simulink model "fig10_70"  (Simulink 7.0)
settings: Solver=ode23s  SolverMode=SingleTasking  StartTime=0.0  StopTime=100.0  RelTol=1e-3  AbsTol=1e-6
values from neighbouring files (symbols this model uses):
  a = [f, 0*f ... (first row only)    [fig10_18.m]    (also in fig10_19.m; fig10_20.m; fig10_21.m; fig10_22.m)
  b = [g;0*g]    [fig10_18.m]    (also in fig10_19.m; fig10_20.m; fig10_21.m; fig10_22.m)
  c = [0*h, g']    [fig10_18.m]    (also in fig10_19.m; fig10_20.m; fig10_21.m; fig10_22.m)
  k1 = signal1(2)    [f_ptos.m]    (also in fig10_05.m = [0, 0.4]; fig10_06.m = [0 .4]; fig10_15.m = [0:.1:1.4]; fig10_16.m = [0 .4])
undefined symbols (not defined in the file or in its folder): ko, ll
libraries: simulink x1
CloseFcn:
  | ;slview('closediagram',bdroot);
settings Model: Creator=abbas  LastModifiedBy=abbas  ExtModeTrigMode=oneshot  ExtModeArmWhenConnect=off
settings DataIOCC: LimitDataPoints=off
settings OptimizationCC: BlockReduction=off  BooleanDataType=off  InlineInvariantSignals=on
settings DebuggingCC: SaveWithParameterizedLinksMsg=none  SignalResolutionControl=TryResolveAllWithWarning  SolverPrmCheckMsg=none  MultiTaskDSMMsg=warning  MultiTaskCondExecSysMsg=none  StrictBusMsg=None
settings HardwareCC: TargetUnknown=on
settings RTWCC: IncludeERTFirstTime=on
settings GRTTargetCC: TargetFcnLib=ansi_tfl_tmw.mat  ModelReferenceCompliant=off  CompOptLevelCompliant=off  MatFileLogging=off

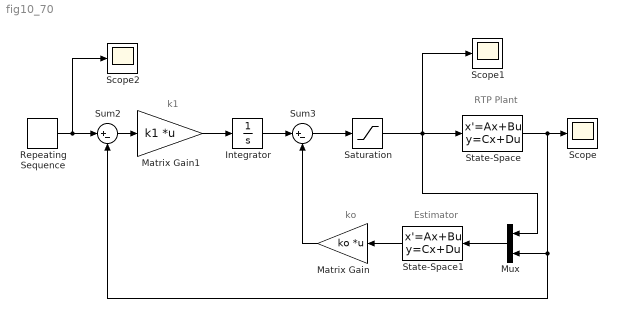
== system fig10_70 ==
  note: ko
  note: k1
  note: Estimator
  note: RTP Plant
  Integrator : Integrator
  Matrix Gain : Gain  Orientation=left  Gain=ko  Multiplication=Matrix(K*u)  ParameterDataType=sfix(16)  ParameterScaling=2^0  OutDataType=sfix(16)  OutScaling=2^0  SaturateOnIntegerOverflow=on
  Matrix Gain1 : Gain  Gain=k1  Multiplication=Matrix(K*u)  ParameterDataType=sfix(16)  ParameterScaling=2^0  OutDataType=sfix(16)  OutScaling=2^0  SaturateOnIntegerOverflow=on
  Mux : Mux  Orientation=left  Inputs=2
  Repeating Sequence : simulink/Sources/Repeating Sequence  SystemSampleTime=-1  rep_seq_t=[0:0.1:100]  rep_seq_y=[0:.1:25 25*ones(1,500) 0*ones(1,250)]
  Saturation : Saturate  UpperLimit=20  LowerLimit=-20
  Scope : Scope
      settings: TickLabels=on  DataFormat=Array
  Scope1 : Scope
      settings: TickLabels=on  DataFormat=Array
  Scope2 : Scope
      settings: TickLabels=on  DataFormat=Array
  State-Space : StateSpace  A=a  B=b  C=c  D=[0]
  State-Space1 : StateSpace  Orientation=left  A=a-ll*c  B=[b ll]  C=eye(3)  D=0*ones(3,2)
  Sum2 : Sum  Inputs=|+-  OutDataType=sfix(16)  OutScaling=2^0  SaturateOnIntegerOverflow=on  InputSameDT=on
  Sum3 : Sum  Inputs=|+-  OutDataType=sfix(16)  OutScaling=2^0  SaturateOnIntegerOverflow=on  InputSameDT=on
  wires:
  Matrix Gain1/1 -> Integrator/1
  Integrator/1 -> Sum3/1
  Sum3/1 -> Saturation/1
  Saturation/1 -> State-Space/1, Scope1/1, Mux/1
  Repeating Sequence/1 -> Scope2/1, Sum2/1
  State-Space/1 -> Scope/1, Mux/2, Sum2/2
  State-Space1/1 -> Matrix Gain/1
  Mux/1 -> State-Space1/1
  Matrix Gain/1 -> Sum3/2
  Sum2/1 -> Matrix Gain1/1
